simulink library "inp_BCKP"  (R2021b)
settings: Solver=VariableStepAuto  StartTime=0.0  StopTime=10.0  RelTol=1e-3
undefined symbols (not defined in the file): C_TASK_5MS_S, FALSE, KINP_AcoreReadyToSlp_flg_ovrdflg, KINP_AcoreReadyToSlp_flg_ovrdval, KINP_AllowMovThd_OTA_enum_ovrdflg, KINP_AllowMovThd_OTA_enum_ovrdval, KINP_APSAngleTarget_Deg_ovrdflg, KINP_APSAngleTarget_Deg_ovrdval, KINP_APSDecReq_mps2_ovrdflg, KINP_APSDecReq_mps2_ovrdval, KINP_APSDecReqA_flg_ovrdflg, KINP_APSDecReqA_flg_ovrdval, KINP_APSDFLL_cm_ovrdflg, KINP_APSDFLL_cm_ovrdval, KINP_APSDFLR_cm_ovrdflg, KINP_APSDFLR_cm_ovrdval, KINP_APSDRLL_cm_ovrdflg, KINP_APSDRLL_cm_ovrdval, KINP_APSDRLR_cm_ovrdflg, KINP_APSDRLR_cm_ovrdval, KINP_APSExitCondition_enum_ovrdflg, KINP_APSExitCondition_enum_ovrdval, KINP_APSHWVer_enum_ovrdflg, KINP_APSHWVer_enum_ovrdval, KINP_APSProgressPCT_pct_ovrdflg, KINP_APSProgressPCT_pct_ovrdval, KINP_APSPwrReq_enum_ovrdflg, KINP_APSPwrReq_enum_ovrdval, KINP_APSReq_enum_ovrdflg, KINP_APSReq_enum_ovrdval, KINP_APSRQDisplay_enum_ovrdflg, KINP_APSRQDisplay_enum_ovrdval, KINP_APSRqEPASCtrl_flg_ovrdflg, KINP_APSRqEPASCtrl_flg_ovrdval, KINP_APSShiftPosnReq_enum_ovrdval, KINP_APSShiftPosnReq_enum_ovrflg, KINP_APSSpeedCMD_kph_ovrdval, KINP_APSSpeedCMD_kph_ovrflg, KINP_APSStaSystem_enum_ovrdflg, KINP_APSStaSystem_enum_ovrdval, KINP_APSSWVer_enum_ovrdflg, KINP_APSSWVer_enum_ovrdval, KINP_APSVMCReqA_flg_ovrdval, KINP_APSVMCReqA_flg_ovrflg, KINP_APSVRqEPASCtrl_flg_ovrdflg, KINP_APSVRqEPASCtrl_flg_ovrdval, KINP_AuxBattVolmV_mV_ovrdflg, KINP_AuxBattVolmV_mV_ovrdval, KINP_BTConnectSta_enum_ovrdflg, KINP_BTConnectSta_enum_ovrdval, KINP_CAASSta_enum_ovrdflg, KINP_CAASSta_enum_ovrdval, KINP_CAASVMCReqA_flg_ovrdval, KINP_CAASVMCReqA_flg_ovrflg, KINP_CAN1BusOff_flg_ovrdflg, KINP_CAN1BusOff_flg_ovrdval, KINP_CAN2BusOff_flg_ovrdflg, KINP_CAN2BusOff_flg_ovrdval, KINP_CAN3BusOff_flg_ovrdflg, KINP_CAN3BusOff_flg_ovrdval ... (+158)
libraries: FVT_lib x144, hcu_lib x1
(part 7 of 8)

== system inp_BCKP/INP/CAN3/SignalCheck/B2TM_Info ==
  BHAL_outputs : Inport
  inp_CanValid_bus : Inport  Port=2
  B2THVRlySta : FVT_lib/inp/can_signal_template  SystemSampleTime=-1  VariantActivationTime=update diagram  Latency=0  AutoFrameSizeCalculation=off
      link override defval: Value=KINP_B2THVRlySta_enum_defval
      link override ovrdflg: Value=KINP_B2THVRlySta_enum_ovrdflg
      link override ovrdval: Value=KINP_B2THVRlySta_enum_ovrdval
  Terminator_1 : Terminator
  True_VHAL_B2THVRlySta_enum : Constant  Value=TRUE  OutDataTypeStr=boolean
  slr1_1 : BusSelector  OutputSignals=VINP_CANMsgValidB2TMInfo_flg
  slr_VHAL_B2THVRlySta_enum : BusSelector  OutputSignals=VHAL_B2THVRlySta_enum
  VINP_B2THVRlySta_enum : Outport
  wires:
  BHAL_outputs/1 -> [BHAL_outputs]
  inp_CanValid_bus/1 -> [inp_CanValid_bus]
  [BHAL_outputs] -> slr_VHAL_B2THVRlySta_enum/1
  slr_VHAL_B2THVRlySta_enum/1 -> B2THVRlySta/1  "<VHAL_B2THVRlySta_enum>"
  True_VHAL_B2THVRlySta_enum/1 -> B2THVRlySta/2
  [inp_CanValid_bus] -> slr1_1/1
  slr1_1/1 -> B2THVRlySta/3  "<VINP_CANMsgValidB2TMInfo_flg>"
  B2THVRlySta/1 -> VINP_B2THVRlySta_enum/1  "VINP_B2THVRlySta_enum"
  B2THVRlySta/2 -> Terminator_1/1

== system inp_BCKP/INP/CAN3/SignalCheck/B2V_BattInfo1 ==
  BHAL_outputs : Inport
  inp_CanValid_bus : Inport  Port=2
  B2VBI1BattType : FVT_lib/inp/can_signal_template  SystemSampleTime=-1  VariantActivationTime=update diagram  Latency=0  AutoFrameSizeCalculation=off
      link override defval: Value=KINP_B2VBI1BattType_enum_defval
      link override ovrdflg: Value=KINP_B2VBI1BattType_enum_ovrdflg
      link override ovrdval: Value=KINP_B2VBI1BattType_enum_ovrdval
  Terminator_1 : Terminator
  True_VHAL_B2VBI1BattType_enum : Constant  Value=TRUE  OutDataTypeStr=boolean
  slr1_1 : BusSelector  OutputSignals=VINP_CANMsgValidB2VBattInfo1_flg
  slr_VHAL_B2VBI1BattType_enum : BusSelector  OutputSignals=VHAL_B2VBI1BattType_enum
  VINP_B2VBI1BattType_enum : Outport
  wires:
  BHAL_outputs/1 -> [BHAL_outputs]
  inp_CanValid_bus/1 -> [inp_CanValid_bus]
  [BHAL_outputs] -> slr_VHAL_B2VBI1BattType_enum/1
  slr_VHAL_B2VBI1BattType_enum/1 -> B2VBI1BattType/1  "<VHAL_B2VBI1BattType_enum>"
  True_VHAL_B2VBI1BattType_enum/1 -> B2VBI1BattType/2
  [inp_CanValid_bus] -> slr1_1/1
  slr1_1/1 -> B2VBI1BattType/3  "<VINP_CANMsgValidB2VBattInfo1_flg>"
  B2VBI1BattType/1 -> VINP_B2VBI1BattType_enum/1  "VINP_B2VBI1BattType_enum"
  B2VBI1BattType/2 -> Terminator_1/1

== system inp_BCKP/INP/CAN3/SignalCheck/B2V_CurrentLimit ==
  BHAL_outputs : Inport
  inp_CanValid_bus : Inport  Port=2
  B2VAPlsDischgCurr : FVT_lib/inp/can_signal_template  SystemSampleTime=-1  VariantActivationTime=update diagram  Latency=0  AutoFrameSizeCalculation=off
      link override defval: Value=KINP_B2VAPlsDischgCurr_A_defval
      link override ovrdflg: Value=KINP_B2VAPlsDischgCurr_A_ovrdflg
      link override ovrdval: Value=KINP_B2VAPlsDischgCurr_A_ovrdval
  Terminator_1 : Terminator
  True_VHAL_B2VAPlsDischgCurr_A : Constant  Value=TRUE  OutDataTypeStr=boolean
  slr1_1 : BusSelector  OutputSignals=VINP_CANMsgValidB2VCurrentLimit_flg
  slr_VHAL_B2VAPlsDischgCurr_A : BusSelector  OutputSignals=VHAL_B2VAPlsDischgCurr_A
  VINP_B2VAPlsDischgCurr_A : Outport
  wires:
  BHAL_outputs/1 -> [BHAL_outputs]
  inp_CanValid_bus/1 -> [inp_CanValid_bus]
  [BHAL_outputs] -> slr_VHAL_B2VAPlsDischgCurr_A/1
  slr_VHAL_B2VAPlsDischgCurr_A/1 -> B2VAPlsDischgCurr/1  "<VHAL_B2VAPlsDischgCurr_A>"
  True_VHAL_B2VAPlsDischgCurr_A/1 -> B2VAPlsDischgCurr/2
  [inp_CanValid_bus] -> slr1_1/1
  slr1_1/1 -> B2VAPlsDischgCurr/3  "<VINP_CANMsgValidB2VCurrentLimit_flg>"
  B2VAPlsDischgCurr/1 -> VINP_B2VAPlsDischgCurr_A/1  "VINP_B2VAPlsDischgCurr_A"
  B2VAPlsDischgCurr/2 -> Terminator_1/1

== system inp_BCKP/INP/CAN3/SignalCheck/B2V_Fult1_32960 ==
  BHAL_outputs : Inport
  inp_CanValid_bus : Inport  Port=2
  B2VHVILFault : FVT_lib/inp/can_signal_template  SystemSampleTime=-1  VariantActivationTime=update diagram  Latency=0  AutoFrameSizeCalculation=off
      link override defval: Value=KINP_B2VHVILFault_flg_defval
      link override ovrdflg: Value=KINP_B2VHVILFault_flg_ovrdflg
      link override ovrdval: Value=KINP_B2VHVILFault_flg_ovrdval
  Terminator_1 : Terminator
  True_VHAL_B2VHVILFault_flg : Constant  Value=TRUE  OutDataTypeStr=boolean
  slr1_1 : BusSelector  OutputSignals=VINP_CANMsgValidB2VFult132960_flg
  slr_VHAL_B2VHVILFault_flg : BusSelector  OutputSignals=VHAL_B2VHVILFault_flg
  VINP_B2VHVILFault_flg : Outport
  wires:
  BHAL_outputs/1 -> [BHAL_outputs]
  inp_CanValid_bus/1 -> [inp_CanValid_bus]
  [BHAL_outputs] -> slr_VHAL_B2VHVILFault_flg/1
  slr_VHAL_B2VHVILFault_flg/1 -> B2VHVILFault/1  "<VHAL_B2VHVILFault_flg>"
  True_VHAL_B2VHVILFault_flg/1 -> B2VHVILFault/2
  [inp_CanValid_bus] -> slr1_1/1
  slr1_1/1 -> B2VHVILFault/3  "<VINP_CANMsgValidB2VFult132960_flg>"
  B2VHVILFault/1 -> VINP_B2VHVILFault_flg/1  "VINP_B2VHVILFault_flg"
  B2VHVILFault/2 -> Terminator_1/1

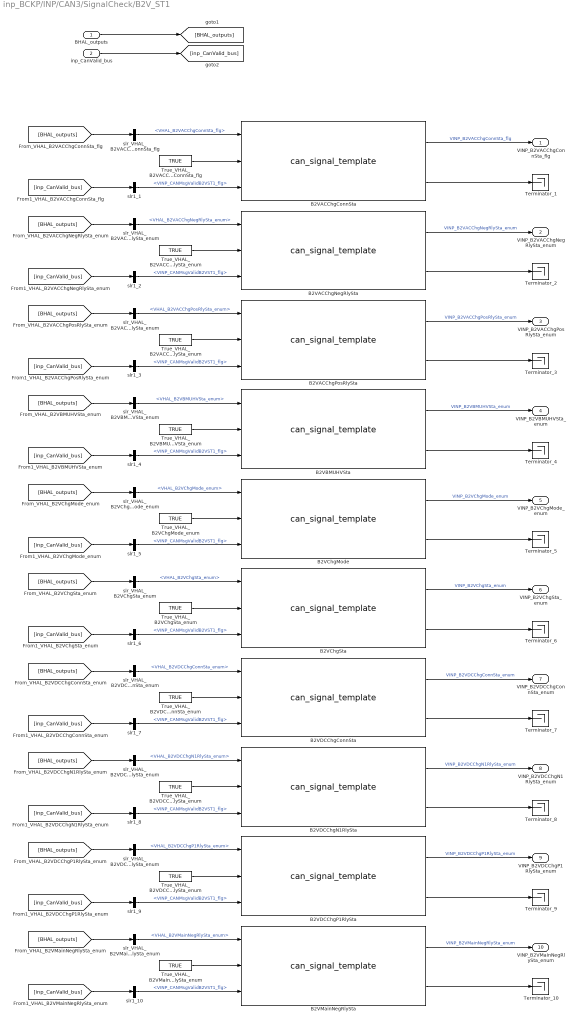
== system inp_BCKP/INP/CAN3/SignalCheck/B2V_ST1 ==
  BHAL_outputs : Inport
  inp_CanValid_bus : Inport  Port=2
  B2VACChgConnSta : FVT_lib/inp/can_signal_template  SystemSampleTime=-1  VariantActivationTime=update diagram  Latency=0  AutoFrameSizeCalculation=off
      link override defval: Value=KINP_B2VACChgConnSta_flg_defval
      link override ovrdflg: Value=KINP_B2VACChgConnSta_flg_ovrdflg
      link override ovrdval: Value=KINP_B2VACChgConnSta_flg_ovrdval
  B2VACChgNegRlySta : FVT_lib/inp/can_signal_template  SystemSampleTime=-1  VariantActivationTime=update diagram  Latency=0  AutoFrameSizeCalculation=off
      link override defval: Value=KINP_B2VACChgNegRlySta_enum_defval
      link override ovrdflg: Value=KINP_B2VACChgNegRlySta_enum_ovrdflg
      link override ovrdval: Value=KINP_B2VACChgNegRlySta_enum_ovrdval
  B2VACChgPosRlySta : FVT_lib/inp/can_signal_template  SystemSampleTime=-1  VariantActivationTime=update diagram  Latency=0  AutoFrameSizeCalculation=off
      link override defval: Value=KINP_B2VACChgPosRlySta_enum_defval
      link override ovrdflg: Value=KINP_B2VACChgPosRlySta_enum_ovrdflg
      link override ovrdval: Value=KINP_B2VACChgPosRlySta_enum_ovrdval
  B2VBMUHVSta : FVT_lib/inp/can_signal_template  SystemSampleTime=-1  VariantActivationTime=update diagram  Latency=0  AutoFrameSizeCalculation=off
      link override defval: Value=KINP_B2VBMUHVSta_enum_defval
      link override ovrdflg: Value=KINP_B2VBMUHVSta_enum_ovrdflg
      link override ovrdval: Value=KINP_B2VBMUHVSta_enum_ovrdval
  B2VChgMode : FVT_lib/inp/can_signal_template  SystemSampleTime=-1  VariantActivationTime=update diagram  Latency=0  AutoFrameSizeCalculation=off
      link override defval: Value=KINP_B2VChgMode_enum_defval
      link override ovrdflg: Value=KINP_B2VChgMode_enum_ovrdflg
      link override ovrdval: Value=KINP_B2VChgMode_enum_ovrdval
  B2VChgSta : FVT_lib/inp/can_signal_template  SystemSampleTime=-1  VariantActivationTime=update diagram  Latency=0  AutoFrameSizeCalculation=off
      link override defval: Value=KINP_B2VChgSta_enum_defval
      link override ovrdflg: Value=KINP_B2VChgSta_enum_ovrdflg
      link override ovrdval: Value=KINP_B2VChgSta_enum_ovrdval
  B2VDCChgConnSta : FVT_lib/inp/can_signal_template  SystemSampleTime=-1  VariantActivationTime=update diagram  Latency=0  AutoFrameSizeCalculation=off
      link override defval: Value=KINP_B2VDCChgConnSta_enum_defval
      link override ovrdflg: Value=KINP_B2VDCChgConnSta_enum_ovrdflg
      link override ovrdval: Value=KINP_B2VDCChgConnSta_enum_ovrdval
  B2VDCChgN1RlySta : FVT_lib/inp/can_signal_template  SystemSampleTime=-1  VariantActivationTime=update diagram  Latency=0  AutoFrameSizeCalculation=off
      link override defval: Value=KINP_B2VDCChgN1RlySta_enum_defval
      link override ovrdflg: Value=KINP_B2VDCChgN1RlySta_enum_ovrdflg
      link override ovrdval: Value=KINP_B2VDCChgN1RlySta_enum_ovrdval
  B2VDCChgP1RlySta : FVT_lib/inp/can_signal_template  SystemSampleTime=-1  VariantActivationTime=update diagram  Latency=0  AutoFrameSizeCalculation=off
      link override defval: Value=KINP_B2VDCChgP1RlySta_enum_defval
      link override ovrdflg: Value=KINP_B2VDCChgP1RlySta_enum_ovrdflg
      link override ovrdval: Value=KINP_B2VDCChgP1RlySta_enum_ovrdval
  B2VMainNegRlySta : FVT_lib/inp/can_signal_template  SystemSampleTime=-1  VariantActivationTime=update diagram  Latency=0  AutoFrameSizeCalculation=off
      link override defval: Value=KINP_B2VMainNegRlySta_enum_defval
      link override ovrdflg: Value=KINP_B2VMainNegRlySta_enum_ovrdflg
      link override ovrdval: Value=KINP_B2VMainNegRlySta_enum_ovrdval
  Terminator_{1..10} (10 alike) : Terminator
  True_VHAL_B2VACChgConnSta_flg : Constant  Value=TRUE  OutDataTypeStr=boolean
  True_VHAL_B2VACChgNegRlySta_enum : Constant  Value=TRUE  OutDataTypeStr=boolean
  True_VHAL_B2VACChgPosRlySta_enum : Constant  Value=TRUE  OutDataTypeStr=boolean
  True_VHAL_B2VBMUHVSta_enum : Constant  Value=TRUE  OutDataTypeStr=boolean
  True_VHAL_B2VChgMode_enum : Constant  Value=TRUE  OutDataTypeStr=boolean
  True_VHAL_B2VChgSta_enum : Constant  Value=TRUE  OutDataTypeStr=boolean
  True_VHAL_B2VDCChgConnSta_enum : Constant  Value=TRUE  OutDataTypeStr=boolean
  True_VHAL_B2VDCChgN1RlySta_enum : Constant  Value=TRUE  OutDataTypeStr=boolean
  True_VHAL_B2VDCChgP1RlySta_enum : Constant  Value=TRUE  OutDataTypeStr=boolean
  True_VHAL_B2VMainNegRlySta_enum : Constant  Value=TRUE  OutDataTypeStr=boolean
  slr1_{1..10} (10 alike) : BusSelector  OutputSignals=VINP_CANMsgValidB2VST1_flg
  slr_VHAL_B2VACChgConnSta_flg : BusSelector  OutputSignals=VHAL_B2VACChgConnSta_flg
  slr_VHAL_B2VACChgNegRlySta_enum : BusSelector  OutputSignals=VHAL_B2VACChgNegRlySta_enum
  slr_VHAL_B2VACChgPosRlySta_enum : BusSelector  OutputSignals=VHAL_B2VACChgPosRlySta_enum
  slr_VHAL_B2VBMUHVSta_enum : BusSelector  OutputSignals=VHAL_B2VBMUHVSta_enum
  slr_VHAL_B2VChgMode_enum : BusSelector  OutputSignals=VHAL_B2VChgMode_enum
  slr_VHAL_B2VChgSta_enum : BusSelector  OutputSignals=VHAL_B2VChgSta_enum
  slr_VHAL_B2VDCChgConnSta_enum : BusSelector  OutputSignals=VHAL_B2VDCChgConnSta_enum
  slr_VHAL_B2VDCChgN1RlySta_enum : BusSelector  OutputSignals=VHAL_B2VDCChgN1RlySta_enum
  slr_VHAL_B2VDCChgP1RlySta_enum : BusSelector  OutputSignals=VHAL_B2VDCChgP1RlySta_enum
  slr_VHAL_B2VMainNegRlySta_enum : BusSelector  OutputSignals=VHAL_B2VMainNegRlySta_enum
  VINP_B2VACChgConnSta_flg : Outport
  VINP_B2VACChgNegRlySta_enum : Outport  Port=2
  VINP_B2VACChgPosRlySta_enum : Outport  Port=3
  VINP_B2VBMUHVSta_enum : Outport  Port=4
  VINP_B2VChgMode_enum : Outport  Port=5
  VINP_B2VChgSta_enum : Outport  Port=6
  VINP_B2VDCChgConnSta_enum : Outport  Port=7
  VINP_B2VDCChgN1RlySta_enum : Outport  Port=8
  VINP_B2VDCChgP1RlySta_enum : Outport  Port=9
  VINP_B2VMainNegRlySta_enum : Outport  Port=10
  wires:
  BHAL_outputs/1 -> [BHAL_outputs]
  inp_CanValid_bus/1 -> [inp_CanValid_bus]
  [BHAL_outputs] -> slr_VHAL_B2VACChgConnSta_flg/1
  slr_VHAL_B2VACChgConnSta_flg/1 -> B2VACChgConnSta/1  "<VHAL_B2VACChgConnSta_flg>"
  True_VHAL_B2VACChgConnSta_flg/1 -> B2VACChgConnSta/2
  [inp_CanValid_bus] -> slr1_1/1
  slr1_1/1 -> B2VACChgConnSta/3  "<VINP_CANMsgValidB2VST1_flg>"
  B2VACChgConnSta/1 -> VINP_B2VACChgConnSta_flg/1  "VINP_B2VACChgConnSta_flg"
  B2VACChgConnSta/2 -> Terminator_1/1
  [BHAL_outputs] -> slr_VHAL_B2VACChgNegRlySta_enum/1
  slr_VHAL_B2VACChgNegRlySta_enum/1 -> B2VACChgNegRlySta/1  "<VHAL_B2VACChgNegRlySta_enum>"
  True_VHAL_B2VACChgNegRlySta_enum/1 -> B2VACChgNegRlySta/2
  [inp_CanValid_bus] -> slr1_2/1
  slr1_2/1 -> B2VACChgNegRlySta/3  "<VINP_CANMsgValidB2VST1_flg>"
  B2VACChgNegRlySta/1 -> VINP_B2VACChgNegRlySta_enum/1  "VINP_B2VACChgNegRlySta_enum"
  B2VACChgNegRlySta/2 -> Terminator_2/1
  [BHAL_outputs] -> slr_VHAL_B2VACChgPosRlySta_enum/1
  slr_VHAL_B2VACChgPosRlySta_enum/1 -> B2VACChgPosRlySta/1  "<VHAL_B2VACChgPosRlySta_enum>"
  True_VHAL_B2VACChgPosRlySta_enum/1 -> B2VACChgPosRlySta/2
  [inp_CanValid_bus] -> slr1_3/1
  slr1_3/1 -> B2VACChgPosRlySta/3  "<VINP_CANMsgValidB2VST1_flg>"
  B2VACChgPosRlySta/1 -> VINP_B2VACChgPosRlySta_enum/1  "VINP_B2VACChgPosRlySta_enum"
  B2VACChgPosRlySta/2 -> Terminator_3/1
  [BHAL_outputs] -> slr_VHAL_B2VBMUHVSta_enum/1
  slr_VHAL_B2VBMUHVSta_enum/1 -> B2VBMUHVSta/1  "<VHAL_B2VBMUHVSta_enum>"
  True_VHAL_B2VBMUHVSta_enum/1 -> B2VBMUHVSta/2
  [inp_CanValid_bus] -> slr1_4/1
  slr1_4/1 -> B2VBMUHVSta/3  "<VINP_CANMsgValidB2VST1_flg>"
  B2VBMUHVSta/1 -> VINP_B2VBMUHVSta_enum/1  "VINP_B2VBMUHVSta_enum"
  B2VBMUHVSta/2 -> Terminator_4/1
  [BHAL_outputs] -> slr_VHAL_B2VChgMode_enum/1
  slr_VHAL_B2VChgMode_enum/1 -> B2VChgMode/1  "<VHAL_B2VChgMode_enum>"
  True_VHAL_B2VChgMode_enum/1 -> B2VChgMode/2
  [inp_CanValid_bus] -> slr1_5/1
  slr1_5/1 -> B2VChgMode/3  "<VINP_CANMsgValidB2VST1_flg>"
  B2VChgMode/1 -> VINP_B2VChgMode_enum/1  "VINP_B2VChgMode_enum"
  B2VChgMode/2 -> Terminator_5/1
  [BHAL_outputs] -> slr_VHAL_B2VChgSta_enum/1
  slr_VHAL_B2VChgSta_enum/1 -> B2VChgSta/1  "<VHAL_B2VChgSta_enum>"
  True_VHAL_B2VChgSta_enum/1 -> B2VChgSta/2
  [inp_CanValid_bus] -> slr1_6/1
  slr1_6/1 -> B2VChgSta/3  "<VINP_CANMsgValidB2VST1_flg>"
  B2VChgSta/1 -> VINP_B2VChgSta_enum/1  "VINP_B2VChgSta_enum"
  B2VChgSta/2 -> Terminator_6/1
  [BHAL_outputs] -> slr_VHAL_B2VDCChgConnSta_enum/1
  slr_VHAL_B2VDCChgConnSta_enum/1 -> B2VDCChgConnSta/1  "<VHAL_B2VDCChgConnSta_enum>"
  True_VHAL_B2VDCChgConnSta_enum/1 -> B2VDCChgConnSta/2
  [inp_CanValid_bus] -> slr1_7/1
  slr1_7/1 -> B2VDCChgConnSta/3  "<VINP_CANMsgValidB2VST1_flg>"
  B2VDCChgConnSta/1 -> VINP_B2VDCChgConnSta_enum/1  "VINP_B2VDCChgConnSta_enum"
  B2VDCChgConnSta/2 -> Terminator_7/1
  [BHAL_outputs] -> slr_VHAL_B2VDCChgN1RlySta_enum/1
  slr_VHAL_B2VDCChgN1RlySta_enum/1 -> B2VDCChgN1RlySta/1  "<VHAL_B2VDCChgN1RlySta_enum>"
  True_VHAL_B2VDCChgN1RlySta_enum/1 -> B2VDCChgN1RlySta/2
  [inp_CanValid_bus] -> slr1_8/1
  slr1_8/1 -> B2VDCChgN1RlySta/3  "<VINP_CANMsgValidB2VST1_flg>"
  B2VDCChgN1RlySta/1 -> VINP_B2VDCChgN1RlySta_enum/1  "VINP_B2VDCChgN1RlySta_enum"
  B2VDCChgN1RlySta/2 -> Terminator_8/1
  [BHAL_outputs] -> slr_VHAL_B2VDCChgP1RlySta_enum/1
  slr_VHAL_B2VDCChgP1RlySta_enum/1 -> B2VDCChgP1RlySta/1  "<VHAL_B2VDCChgP1RlySta_enum>"
  True_VHAL_B2VDCChgP1RlySta_enum/1 -> B2VDCChgP1RlySta/2
  [inp_CanValid_bus] -> slr1_9/1
  slr1_9/1 -> B2VDCChgP1RlySta/3  "<VINP_CANMsgValidB2VST1_flg>"
  B2VDCChgP1RlySta/1 -> VINP_B2VDCChgP1RlySta_enum/1  "VINP_B2VDCChgP1RlySta_enum"
  B2VDCChgP1RlySta/2 -> Terminator_9/1
  [BHAL_outputs] -> slr_VHAL_B2VMainNegRlySta_enum/1
  slr_VHAL_B2VMainNegRlySta_enum/1 -> B2VMainNegRlySta/1  "<VHAL_B2VMainNegRlySta_enum>"
  True_VHAL_B2VMainNegRlySta_enum/1 -> B2VMainNegRlySta/2
  [inp_CanValid_bus] -> slr1_10/1
  slr1_10/1 -> B2VMainNegRlySta/3  "<VINP_CANMsgValidB2VST1_flg>"
  B2VMainNegRlySta/1 -> VINP_B2VMainNegRlySta_enum/1  "VINP_B2VMainNegRlySta_enum"
  B2VMainNegRlySta/2 -> Terminator_10/1

== system inp_BCKP/INP/CAN3/SignalCheck/B2V_ST2 ==
  BHAL_outputs : Inport
  inp_CanValid_bus : Inport  Port=2
  B2VFaultCode : FVT_lib/inp/can_signal_template  SystemSampleTime=-1  VariantActivationTime=update diagram  Latency=0  AutoFrameSizeCalculation=off
      link override defval: Value=KINP_B2VFaultCode_enum_defval
      link override ovrdflg: Value=KINP_B2VFaultCode_enum_ovrdflg
      link override ovrdval: Value=KINP_B2VFaultCode_enum_ovrdval
  B2VRqHVPwrOff : FVT_lib/inp/can_signal_template  SystemSampleTime=-1  VariantActivationTime=update diagram  Latency=0  AutoFrameSizeCalculation=off
      link override defval: Value=KINP_B2VRqHVPwrOff_enum_defval
      link override ovrdflg: Value=KINP_B2VRqHVPwrOff_enum_ovrdflg
      link override ovrdval: Value=KINP_B2VRqHVPwrOff_enum_ovrdval
  B2VSOC : FVT_lib/inp/can_signal_template  SystemSampleTime=-1  VariantActivationTime=update diagram  Latency=0  AutoFrameSizeCalculation=off
      link override defval: Value=KINP_B2VSOC_pct_defval
      link override ovrdflg: Value=KINP_B2VSOC_pct_ovrdflg
      link override ovrdval: Value=KINP_B2VSOC_pct_ovrdval
  Terminator_1 : Terminator
  Terminator_2 : Terminator
  Terminator_3 : Terminator
  True_VHAL_B2VFaultCode_enum : Constant  Value=TRUE  OutDataTypeStr=boolean
  True_VHAL_B2VRqHVPwrOff_enum : Constant  Value=TRUE  OutDataTypeStr=boolean
  True_VHAL_B2VSOC_pct : Constant  Value=TRUE  OutDataTypeStr=boolean
  slr1_1 : BusSelector  OutputSignals=VINP_CANMsgValidB2VST2_flg
  slr1_2 : BusSelector  OutputSignals=VINP_CANMsgValidB2VST2_flg
  slr1_3 : BusSelector  OutputSignals=VINP_CANMsgValidB2VST2_flg
  slr_VHAL_B2VFaultCode_enum : BusSelector  OutputSignals=VHAL_B2VFaultCode_enum
  slr_VHAL_B2VRqHVPwrOff_enum : BusSelector  OutputSignals=VHAL_B2VRqHVPwrOff_enum
  slr_VHAL_B2VSOC_pct : BusSelector  OutputSignals=VHAL_B2VSOC_pct
  VINP_B2VFaultCode_enum : Outport
  VINP_B2VRqHVPwrOff_enum : Outport  Port=2
  VINP_B2VSOC_pct : Outport  Port=3
  wires:
  BHAL_outputs/1 -> [BHAL_outputs]
  inp_CanValid_bus/1 -> [inp_CanValid_bus]
  [BHAL_outputs] -> slr_VHAL_B2VFaultCode_enum/1
  slr_VHAL_B2VFaultCode_enum/1 -> B2VFaultCode/1  "<VHAL_B2VFaultCode_enum>"
  True_VHAL_B2VFaultCode_enum/1 -> B2VFaultCode/2
  [inp_CanValid_bus] -> slr1_1/1
  slr1_1/1 -> B2VFaultCode/3  "<VINP_CANMsgValidB2VST2_flg>"
  B2VFaultCode/1 -> VINP_B2VFaultCode_enum/1  "VINP_B2VFaultCode_enum"
  B2VFaultCode/2 -> Terminator_1/1
  [BHAL_outputs] -> slr_VHAL_B2VRqHVPwrOff_enum/1
  slr_VHAL_B2VRqHVPwrOff_enum/1 -> B2VRqHVPwrOff/1  "<VHAL_B2VRqHVPwrOff_enum>"
  True_VHAL_B2VRqHVPwrOff_enum/1 -> B2VRqHVPwrOff/2
  [inp_CanValid_bus] -> slr1_2/1
  slr1_2/1 -> B2VRqHVPwrOff/3  "<VINP_CANMsgValidB2VST2_flg>"
  B2VRqHVPwrOff/1 -> VINP_B2VRqHVPwrOff_enum/1  "VINP_B2VRqHVPwrOff_enum"
  B2VRqHVPwrOff/2 -> Terminator_2/1
  [BHAL_outputs] -> slr_VHAL_B2VSOC_pct/1
  slr_VHAL_B2VSOC_pct/1 -> B2VSOC/1  "<VHAL_B2VSOC_pct>"
  True_VHAL_B2VSOC_pct/1 -> B2VSOC/2
  [inp_CanValid_bus] -> slr1_3/1
  slr1_3/1 -> B2VSOC/3  "<VINP_CANMsgValidB2VST2_flg>"
  B2VSOC/1 -> VINP_B2VSOC_pct/1  "VINP_B2VSOC_pct"
  B2VSOC/2 -> Terminator_3/1

== system inp_BCKP/INP/CAN3/SignalCheck/B2V_ST4 ==
  BHAL_outputs : Inport
  inp_CanValid_bus : Inport  Port=2
  B2VMinTempPos : FVT_lib/inp/can_signal_template  SystemSampleTime=-1  VariantActivationTime=update diagram  Latency=0  AutoFrameSizeCalculation=off
      link override defval: Value=KINP_B2VMinTempPos_enum_defval
      link override ovrdflg: Value=KINP_B2VMinTempPos_enum_ovrdflg
      link override ovrdval: Value=KINP_B2VMinTempPos_enum_ovrdval
  Terminator_1 : Terminator
  True_VHAL_B2VMinTempPos_enum : Constant  Value=TRUE  OutDataTypeStr=boolean
  slr1_1 : BusSelector  OutputSignals=VINP_CANMsgValidB2VST4_flg
  slr_VHAL_B2VMinTempPos_enum : BusSelector  OutputSignals=VHAL_B2VMinTempPos_enum
  VINP_B2VMinTempPos_enum : Outport
  wires:
  BHAL_outputs/1 -> [BHAL_outputs]
  inp_CanValid_bus/1 -> [inp_CanValid_bus]
  [BHAL_outputs] -> slr_VHAL_B2VMinTempPos_enum/1
  slr_VHAL_B2VMinTempPos_enum/1 -> B2VMinTempPos/1  "<VHAL_B2VMinTempPos_enum>"
  True_VHAL_B2VMinTempPos_enum/1 -> B2VMinTempPos/2
  [inp_CanValid_bus] -> slr1_1/1
  slr1_1/1 -> B2VMinTempPos/3  "<VINP_CANMsgValidB2VST4_flg>"
  B2VMinTempPos/1 -> VINP_B2VMinTempPos_enum/1  "VINP_B2VMinTempPos_enum"
  B2VMinTempPos/2 -> Terminator_1/1

== system inp_BCKP/INP/CAN3/SignalCheck/B2V_ST5 ==
  BHAL_outputs : Inport
  inp_CanValid_bus : Inport  Port=2
  B2VCellMinVol : FVT_lib/inp/can_signal_template  SystemSampleTime=-1  VariantActivationTime=update diagram  Latency=0  AutoFrameSizeCalculation=off
      link override defval: Value=KINP_B2VCellMinVol_V_defval
      link override ovrdflg: Value=KINP_B2VCellMinVol_V_ovrdflg
      link override ovrdval: Value=KINP_B2VCellMinVol_V_ovrdval
  Terminator_1 : Terminator
  True_VHAL_B2VCellMinVol_V : Constant  Value=TRUE  OutDataTypeStr=boolean
  slr1_1 : BusSelector  OutputSignals=VINP_CANMsgValidB2VST5_flg
  slr_VHAL_B2VCellMinVol_V : BusSelector  OutputSignals=VHAL_B2VCellMinVol_V
  VINP_B2VCellMinVol_V : Outport
  wires:
  BHAL_outputs/1 -> [BHAL_outputs]
  inp_CanValid_bus/1 -> [inp_CanValid_bus]
  [BHAL_outputs] -> slr_VHAL_B2VCellMinVol_V/1
  slr_VHAL_B2VCellMinVol_V/1 -> B2VCellMinVol/1  "<VHAL_B2VCellMinVol_V>"
  True_VHAL_B2VCellMinVol_V/1 -> B2VCellMinVol/2
  [inp_CanValid_bus] -> slr1_1/1
  slr1_1/1 -> B2VCellMinVol/3  "<VINP_CANMsgValidB2VST5_flg>"
  B2VCellMinVol/1 -> VINP_B2VCellMinVol_V/1  "VINP_B2VCellMinVol_V"
  B2VCellMinVol/2 -> Terminator_1/1

== system inp_BCKP/INP/CAN3/SignalCheck/EWP1 ==
  BHAL_outputs : Inport
  inp_CanValid_bus : Inport  Port=2
  EWPPEFault : FVT_lib/inp/can_signal_template  SystemSampleTime=-1  VariantActivationTime=update diagram  Latency=0  AutoFrameSizeCalculation=off
      link override defval: Value=KINP_EWPPEFault_enum_defval
      link override ovrdflg: Value=KINP_EWPPEFault_enum_ovrdflg
      link override ovrdval: Value=KINP_EWPPEFault_enum_ovrdval
  Terminator_1 : Terminator
  True_VHAL_EWPPEFault_enum : Constant  Value=TRUE  OutDataTypeStr=boolean
  slr1_1 : BusSelector  OutputSignals=VINP_CANMsgValidEWP1_flg
  slr_VHAL_EWPPEFault_enum : BusSelector  OutputSignals=VHAL_EWPPEFault_enum
  VINP_EWPPEFault_enum : Outport
  wires:
  BHAL_outputs/1 -> [BHAL_outputs]
  inp_CanValid_bus/1 -> [inp_CanValid_bus]
  [BHAL_outputs] -> slr_VHAL_EWPPEFault_enum/1
  slr_VHAL_EWPPEFault_enum/1 -> EWPPEFault/1  "<VHAL_EWPPEFault_enum>"
  True_VHAL_EWPPEFault_enum/1 -> EWPPEFault/2
  [inp_CanValid_bus] -> slr1_1/1
  slr1_1/1 -> EWPPEFault/3  "<VINP_CANMsgValidEWP1_flg>"
  EWPPEFault/1 -> VINP_EWPPEFault_enum/1  "VINP_EWPPEFault_enum"
  EWPPEFault/2 -> Terminator_1/1

== system inp_BCKP/INP/CAN3/SignalCheck/TM_MCUSta1 ==
  BHAL_outputs : Inport
  inp_CanValid_bus : Inport  Port=2
  AtvDisChgEnFbk : FVT_lib/inp/can_signal_template  SystemSampleTime=-1  VariantActivationTime=update diagram  Latency=0  AutoFrameSizeCalculation=off
      link override defval: Value=KINP_AtvDisChgEnFbk_flg_defval
      link override ovrdflg: Value=KINP_AtvDisChgEnFbk_flg_ovrdflg
      link override ovrdval: Value=KINP_AtvDisChgEnFbk_flg_ovrdval
  MCUCtrlMdSta : FVT_lib/inp/can_signal_template  SystemSampleTime=-1  VariantActivationTime=update diagram  Latency=0  AutoFrameSizeCalculation=off
      link override defval: Value=KINP_MCUCtrlMdSta_enum_defval
      link override ovrdflg: Value=KINP_MCUCtrlMdSta_enum_ovrdflg
      link override ovrdval: Value=KINP_MCUCtrlMdSta_enum_ovrdval
  MCUIGBTEnFbk : FVT_lib/inp/can_signal_template  SystemSampleTime=-1  VariantActivationTime=update diagram  Latency=0  AutoFrameSizeCalculation=off
      link override defval: Value=KINP_MCUIGBTEnFbk_flg_defval
      link override ovrdflg: Value=KINP_MCUIGBTEnFbk_flg_ovrdflg
      link override ovrdval: Value=KINP_MCUIGBTEnFbk_flg_ovrdval
  MotorSpd : FVT_lib/inp/can_signal_template  SystemSampleTime=-1  VariantActivationTime=update diagram  Latency=0  AutoFrameSizeCalculation=off
      link override defval: Value=KINP_MotorSpd_rpm_defval
      link override ovrdflg: Value=KINP_MotorSpd_rpm_ovrdflg
      link override ovrdval: Value=KINP_MotorSpd_rpm_ovrdval
  MotorTrq : FVT_lib/inp/can_signal_template  SystemSampleTime=-1  VariantActivationTime=update diagram  Latency=0  AutoFrameSizeCalculation=off
      link override defval: Value=KINP_MotorTrq_Nm_defval
      link override ovrdflg: Value=KINP_MotorTrq_Nm_ovrdflg
      link override ovrdval: Value=KINP_MotorTrq_Nm_ovrdval
  Terminator_{1..5} (5 alike) : Terminator
  True_VHAL_AtvDisChgEnFbk_flg : Constant  Value=TRUE  OutDataTypeStr=boolean
  True_VHAL_MCUCtrlMdSta_enum : Constant  Value=TRUE  OutDataTypeStr=boolean
  True_VHAL_MCUIGBTEnFbk_flg : Constant  Value=TRUE  OutDataTypeStr=boolean
  True_VHAL_MotorSpd_rpm : Constant  Value=TRUE  OutDataTypeStr=boolean
  True_VHAL_MotorTrq_Nm : Constant  Value=TRUE  OutDataTypeStr=boolean
  slr1_{1..5} (5 alike) : BusSelector  OutputSignals=VINP_CANMsgValidTMMCUSta1_flg
  slr_VHAL_AtvDisChgEnFbk_flg : BusSelector  OutputSignals=VHAL_AtvDisChgEnFbk_flg
  slr_VHAL_MCUCtrlMdSta_enum : BusSelector  OutputSignals=VHAL_MCUCtrlMdSta_enum
  slr_VHAL_MCUIGBTEnFbk_flg : BusSelector  OutputSignals=VHAL_MCUIGBTEnFbk_flg
  slr_VHAL_MotorSpd_rpm : BusSelector  OutputSignals=VHAL_MotorSpd_rpm
  slr_VHAL_MotorTrq_Nm : BusSelector  OutputSignals=VHAL_MotorTrq_Nm
  VINP_AtvDisChgEnFbk_flg : Outport
  VINP_MCUCtrlMdSta_enum : Outport  Port=2
  VINP_MCUIGBTEnFbk_flg : Outport  Port=3
  VINP_MotorSpd_rpm : Outport  Port=4
  VINP_MotorTrq_Nm : Outport  Port=5
  wires:
  BHAL_outputs/1 -> [BHAL_outputs]
  inp_CanValid_bus/1 -> [inp_CanValid_bus]
  [BHAL_outputs] -> slr_VHAL_AtvDisChgEnFbk_flg/1
  slr_VHAL_AtvDisChgEnFbk_flg/1 -> AtvDisChgEnFbk/1  "<VHAL_AtvDisChgEnFbk_flg>"
  True_VHAL_AtvDisChgEnFbk_flg/1 -> AtvDisChgEnFbk/2
  [inp_CanValid_bus] -> slr1_1/1
  slr1_1/1 -> AtvDisChgEnFbk/3  "<VINP_CANMsgValidTMMCUSta1_flg>"
  AtvDisChgEnFbk/1 -> VINP_AtvDisChgEnFbk_flg/1  "VINP_AtvDisChgEnFbk_flg"
  AtvDisChgEnFbk/2 -> Terminator_1/1
  [BHAL_outputs] -> slr_VHAL_MCUCtrlMdSta_enum/1
  slr_VHAL_MCUCtrlMdSta_enum/1 -> MCUCtrlMdSta/1  "<VHAL_MCUCtrlMdSta_enum>"
  True_VHAL_MCUCtrlMdSta_enum/1 -> MCUCtrlMdSta/2
  [inp_CanValid_bus] -> slr1_2/1
  slr1_2/1 -> MCUCtrlMdSta/3  "<VINP_CANMsgValidTMMCUSta1_flg>"
  MCUCtrlMdSta/1 -> VINP_MCUCtrlMdSta_enum/1  "VINP_MCUCtrlMdSta_enum"
  MCUCtrlMdSta/2 -> Terminator_2/1
  [BHAL_outputs] -> slr_VHAL_MCUIGBTEnFbk_flg/1
  slr_VHAL_MCUIGBTEnFbk_flg/1 -> MCUIGBTEnFbk/1  "<VHAL_MCUIGBTEnFbk_flg>"
  True_VHAL_MCUIGBTEnFbk_flg/1 -> MCUIGBTEnFbk/2
  [inp_CanValid_bus] -> slr1_3/1
  slr1_3/1 -> MCUIGBTEnFbk/3  "<VINP_CANMsgValidTMMCUSta1_flg>"
  MCUIGBTEnFbk/1 -> VINP_MCUIGBTEnFbk_flg/1  "VINP_MCUIGBTEnFbk_flg"
  MCUIGBTEnFbk/2 -> Terminator_3/1
  [BHAL_outputs] -> slr_VHAL_MotorSpd_rpm/1
  slr_VHAL_MotorSpd_rpm/1 -> MotorSpd/1  "<VHAL_MotorSpd_rpm>"
  True_VHAL_MotorSpd_rpm/1 -> MotorSpd/2
  [inp_CanValid_bus] -> slr1_4/1
  slr1_4/1 -> MotorSpd/3  "<VINP_CANMsgValidTMMCUSta1_flg>"
  MotorSpd/1 -> VINP_MotorSpd_rpm/1  "VINP_MotorSpd_rpm"
  MotorSpd/2 -> Terminator_4/1
  [BHAL_outputs] -> slr_VHAL_MotorTrq_Nm/1
  slr_VHAL_MotorTrq_Nm/1 -> MotorTrq/1  "<VHAL_MotorTrq_Nm>"
  True_VHAL_MotorTrq_Nm/1 -> MotorTrq/2
  [inp_CanValid_bus] -> slr1_5/1
  slr1_5/1 -> MotorTrq/3  "<VINP_CANMsgValidTMMCUSta1_flg>"
  MotorTrq/1 -> VINP_MotorTrq_Nm/1  "VINP_MotorTrq_Nm"
  MotorTrq/2 -> Terminator_5/1

== system inp_BCKP/INP/CAN3/SignalCheck/TM_MCUSta2 ==
  BHAL_outputs : Inport
  inp_CanValid_bus : Inport  Port=2
  MCUFailGrade : FVT_lib/inp/can_signal_template  SystemSampleTime=-1  VariantActivationTime=update diagram  Latency=0  AutoFrameSizeCalculation=off
      link override defval: Value=KINP_MCUFailGrade_enum_defval
      link override ovrdflg: Value=KINP_MCUFailGrade_enum_ovrdflg
      link override ovrdval: Value=KINP_MCUFailGrade_enum_ovrdval
  MCUTemp : FVT_lib/inp/can_signal_template  SystemSampleTime=-1  VariantActivationTime=update diagram  Latency=0  AutoFrameSizeCalculation=off
      link override defval: Value=KINP_MCUTemp_C_defval
      link override ovrdflg: Value=KINP_MCUTemp_C_ovrdflg
      link override ovrdval: Value=KINP_MCUTemp_C_ovrdval
  Terminator_1 : Terminator
  Terminator_2 : Terminator
  True_VHAL_MCUFailGrade_enum : Constant  Value=TRUE  OutDataTypeStr=boolean
  True_VHAL_MCUTemp_C : Constant  Value=TRUE  OutDataTypeStr=boolean
  slr1_1 : BusSelector  OutputSignals=VINP_CANMsgValidTMMCUSta2_flg
  slr1_2 : BusSelector  OutputSignals=VINP_CANMsgValidTMMCUSta2_flg
  slr_VHAL_MCUFailGrade_enum : BusSelector  OutputSignals=VHAL_MCUFailGrade_enum
  slr_VHAL_MCUTemp_C : BusSelector  OutputSignals=VHAL_MCUTemp_C
  VINP_MCUFailGrade_enum : Outport
  VINP_MCUTemp_C : Outport  Port=2
  wires:
  BHAL_outputs/1 -> [BHAL_outputs]
  inp_CanValid_bus/1 -> [inp_CanValid_bus]
  [BHAL_outputs] -> slr_VHAL_MCUFailGrade_enum/1
  slr_VHAL_MCUFailGrade_enum/1 -> MCUFailGrade/1  "<VHAL_MCUFailGrade_enum>"
  True_VHAL_MCUFailGrade_enum/1 -> MCUFailGrade/2
  [inp_CanValid_bus] -> slr1_1/1
  slr1_1/1 -> MCUFailGrade/3  "<VINP_CANMsgValidTMMCUSta2_flg>"
  MCUFailGrade/1 -> VINP_MCUFailGrade_enum/1  "VINP_MCUFailGrade_enum"
  MCUFailGrade/2 -> Terminator_1/1
  [BHAL_outputs] -> slr_VHAL_MCUTemp_C/1
  slr_VHAL_MCUTemp_C/1 -> MCUTemp/1  "<VHAL_MCUTemp_C>"
  True_VHAL_MCUTemp_C/1 -> MCUTemp/2
  [inp_CanValid_bus] -> slr1_2/1
  slr1_2/1 -> MCUTemp/3  "<VINP_CANMsgValidTMMCUSta2_flg>"
  MCUTemp/1 -> VINP_MCUTemp_C/1  "VINP_MCUTemp_C"
  MCUTemp/2 -> Terminator_2/1

== system inp_BCKP/INP/CAN3/SignalCheck/TM_MCUSta3 ==
  BHAL_outputs : Inport
  inp_CanValid_bus : Inport  Port=2
  MCUDCVol : FVT_lib/inp/can_signal_template  SystemSampleTime=-1  VariantActivationTime=update diagram  Latency=0  AutoFrameSizeCalculation=off
      link override defval: Value=KINP_MCUDCVol_V_defval
      link override ovrdflg: Value=KINP_MCUDCVol_V_ovrdflg
      link override ovrdval: Value=KINP_MCUDCVol_V_ovrdval
  MCUFailCode : FVT_lib/inp/can_signal_template  SystemSampleTime=-1  VariantActivationTime=update diagram  Latency=0  AutoFrameSizeCalculation=off
      link override defval: Value=KINP_MCUFailCode_enum_defval
      link override ovrdflg: Value=KINP_MCUFailCode_enum_ovrdflg
      link override ovrdval: Value=KINP_MCUFailCode_enum_ovrdval
  Terminator_1 : Terminator
  Terminator_2 : Terminator
  True_VHAL_MCUDCVol_V : Constant  Value=TRUE  OutDataTypeStr=boolean
  True_VHAL_MCUFailCode_enum : Constant  Value=TRUE  OutDataTypeStr=boolean
  slr1_1 : BusSelector  OutputSignals=VINP_CANMsgValidTMMCUSta3_flg
  slr1_2 : BusSelector  OutputSignals=VINP_CANMsgValidTMMCUSta3_flg
  slr_VHAL_MCUDCVol_V : BusSelector  OutputSignals=VHAL_MCUDCVol_V
  slr_VHAL_MCUFailCode_enum : BusSelector  OutputSignals=VHAL_MCUFailCode_enum
  VINP_MCUDCVol_V : Outport
  VINP_MCUFailCode_enum : Outport  Port=2
  wires:
  BHAL_outputs/1 -> [BHAL_outputs]
  inp_CanValid_bus/1 -> [inp_CanValid_bus]
  [BHAL_outputs] -> slr_VHAL_MCUDCVol_V/1
  slr_VHAL_MCUDCVol_V/1 -> MCUDCVol/1  "<VHAL_MCUDCVol_V>"
  True_VHAL_MCUDCVol_V/1 -> MCUDCVol/2
  [inp_CanValid_bus] -> slr1_1/1
  slr1_1/1 -> MCUDCVol/3  "<VINP_CANMsgValidTMMCUSta3_flg>"
  MCUDCVol/1 -> VINP_MCUDCVol_V/1  "VINP_MCUDCVol_V"
  MCUDCVol/2 -> Terminator_1/1
  [BHAL_outputs] -> slr_VHAL_MCUFailCode_enum/1
  slr_VHAL_MCUFailCode_enum/1 -> MCUFailCode/1  "<VHAL_MCUFailCode_enum>"
  True_VHAL_MCUFailCode_enum/1 -> MCUFailCode/2
  [inp_CanValid_bus] -> slr1_2/1
  slr1_2/1 -> MCUFailCode/3  "<VINP_CANMsgValidTMMCUSta3_flg>"
  MCUFailCode/1 -> VINP_MCUFailCode_enum/1  "VINP_MCUFailCode_enum"
  MCUFailCode/2 -> Terminator_2/1

== system inp_BCKP/INP/CAN4/SignalCheck/ZFR_CE100_0 ==
  BHAL_outputs : Inport
  inp_CanValid_bus : Inport  Port=2
  Terminator_1 : Terminator
  True_VHAL_ZFRBCMBrakeSta_flg : Constant  Value=TRUE  OutDataTypeStr=boolean
  ZFRBCMBrakeSta : FVT_lib/inp/can_signal_template  SystemSampleTime=-1  VariantActivationTime=update diagram  Latency=0  AutoFrameSizeCalculation=off
      link override defval: Value=KINP_ZFRBCMBrakeSta_flg_defval
      link override ovrdflg: Value=KINP_ZFRBCMBrakeSta_flg_ovrdflg
      link override ovrdval: Value=KINP_ZFRBCMBrakeSta_flg_ovrdval
  slr1_1 : BusSelector  OutputSignals=VINP_CANMsgValidZFRCE1000_flg
  slr_VHAL_ZFRBCMBrakeSta_flg : BusSelector  OutputSignals=VHAL_ZFRBCMBrakeSta_flg
  VINP_ZFRBCMBrakeSta_flg : Outport
  wires:
  BHAL_outputs/1 -> [BHAL_outputs]
  inp_CanValid_bus/1 -> [inp_CanValid_bus]
  [BHAL_outputs] -> slr_VHAL_ZFRBCMBrakeSta_flg/1
  slr_VHAL_ZFRBCMBrakeSta_flg/1 -> ZFRBCMBrakeSta/1  "<VHAL_ZFRBCMBrakeSta_flg>"
  True_VHAL_ZFRBCMBrakeSta_flg/1 -> ZFRBCMBrakeSta/2
  [inp_CanValid_bus] -> slr1_1/1
  slr1_1/1 -> ZFRBCMBrakeSta/3  "<VINP_CANMsgValidZFRCE1000_flg>"
  ZFRBCMBrakeSta/1 -> VINP_ZFRBCMBrakeSta_flg/1  "VINP_ZFRBCMBrakeSta_flg"
  ZFRBCMBrakeSta/2 -> Terminator_1/1

== system inp_BCKP/INP/CAN4/SignalCheck/ZRR_CE100_0 ==
  BHAL_outputs : Inport
  inp_CanValid_bus : Inport  Port=2
  Terminator_1 : Terminator
  True_VHAL_ZRRBCMAllDoorSta_enum : Constant  Value=TRUE  OutDataTypeStr=boolean
  ZRRBCMAllDoorSta : FVT_lib/inp/can_signal_template  SystemSampleTime=-1  VariantActivationTime=update diagram  Latency=0  AutoFrameSizeCalculation=off
      link override defval: Value=KINP_ZRRBCMAllDoorSta_enum_defval
      link override ovrdflg: Value=KINP_ZRRBCMAllDoorSta_enum_ovrdflg
      link override ovrdval: Value=KINP_ZRRBCMAllDoorSta_enum_ovrdval
  slr1_1 : BusSelector  OutputSignals=VINP_CANMsgValidZRRCE1000_flg
  slr_VHAL_ZRRBCMAllDoorSta_enum : BusSelector  OutputSignals=VHAL_ZRRBCMAllDoorSta_enum
  VINP_ZRRBCMAllDoorSta_enum : Outport
  wires:
  BHAL_outputs/1 -> [BHAL_outputs]
  inp_CanValid_bus/1 -> [inp_CanValid_bus]
  [BHAL_outputs] -> slr_VHAL_ZRRBCMAllDoorSta_enum/1
  slr_VHAL_ZRRBCMAllDoorSta_enum/1 -> ZRRBCMAllDoorSta/1  "<VHAL_ZRRBCMAllDoorSta_enum>"
  True_VHAL_ZRRBCMAllDoorSta_enum/1 -> ZRRBCMAllDoorSta/2
  [inp_CanValid_bus] -> slr1_1/1
  slr1_1/1 -> ZRRBCMAllDoorSta/3  "<VINP_CANMsgValidZRRCE1000_flg>"
  ZRRBCMAllDoorSta/1 -> VINP_ZRRBCMAllDoorSta_enum/1  "VINP_ZRRBCMAllDoorSta_enum"
  ZRRBCMAllDoorSta/2 -> Terminator_1/1

== system inp_BCKP/INP/CAN4/SignalCheck/ZRR_CE100_1 ==
  BHAL_outputs : Inport
  inp_CanValid_bus : Inport  Port=2
  Terminator_1 : Terminator
  True_VHAL_ZRRBCMPLampSta_flg : Constant  Value=TRUE  OutDataTypeStr=boolean
  ZRRBCMPLampSta : FVT_lib/inp/can_signal_template  SystemSampleTime=-1  VariantActivationTime=update diagram  Latency=0  AutoFrameSizeCalculation=off
      link override defval: Value=KINP_ZRRBCMPLampSta_flg_defval
      link override ovrdflg: Value=KINP_ZRRBCMPLampSta_flg_ovrdflg
      link override ovrdval: Value=KINP_ZRRBCMPLampSta_flg_ovrdval
  slr1_1 : BusSelector  OutputSignals=VINP_CANMsgValidZRRCE1001_flg
  slr_VHAL_ZRRBCMPLampSta_flg : BusSelector  OutputSignals=VHAL_ZRRBCMPLampSta_flg
  VINP_ZRRBCMPLampSta_flg : Outport
  wires:
  BHAL_outputs/1 -> [BHAL_outputs]
  inp_CanValid_bus/1 -> [inp_CanValid_bus]
  [BHAL_outputs] -> slr_VHAL_ZRRBCMPLampSta_flg/1
  slr_VHAL_ZRRBCMPLampSta_flg/1 -> ZRRBCMPLampSta/1  "<VHAL_ZRRBCMPLampSta_flg>"
  True_VHAL_ZRRBCMPLampSta_flg/1 -> ZRRBCMPLampSta/2
  [inp_CanValid_bus] -> slr1_1/1
  slr1_1/1 -> ZRRBCMPLampSta/3  "<VINP_CANMsgValidZRRCE1001_flg>"
  ZRRBCMPLampSta/1 -> VINP_ZRRBCMPLampSta_flg/1  "VINP_ZRRBCMPLampSta_flg"
  ZRRBCMPLampSta/2 -> Terminator_1/1
